simulink model "ex4_s1_simulink"  (R2014b)
settings: Solver=ode45  StartTime=0.0  StopTime=time  RelTol=1e-3
values from neighbouring files (symbols this model uses):
  C = 10e-6    (= 1e-05)    [ex4.m]
  G1 = 1/(R1*C*s + 1)    [ex4.m]
  R1 = 200    [ex4.m]
  R2 = 200    [ex4.m]
undefined symbols (not defined in the file or in its folder): S2
settings Model: Creator=gabras  LastModifiedBy=gabras

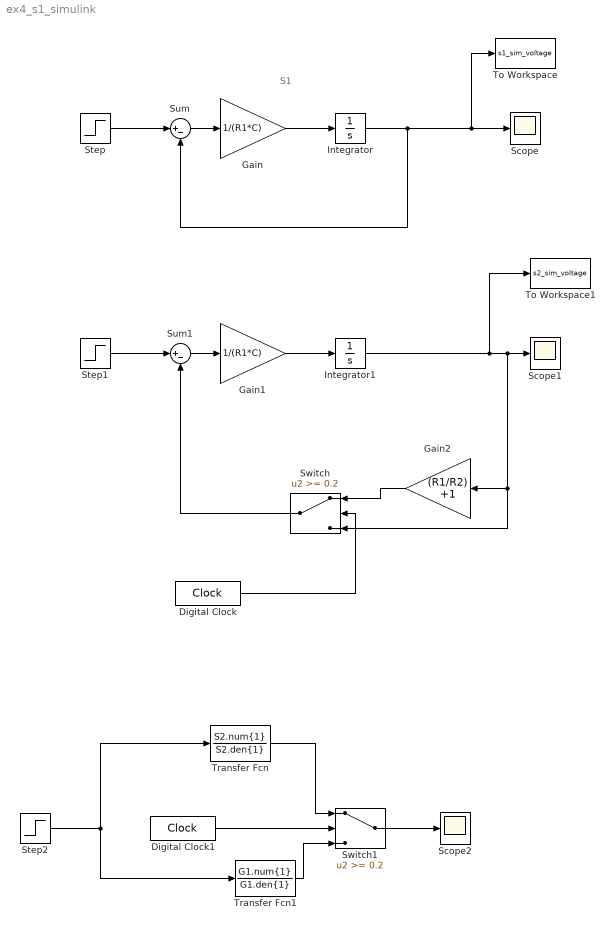
== system ex4_s1_simulink ==
  note: S1
  Digital Clock : DigitalClock  SampleTime=0.1
  Digital Clock1 : DigitalClock  SampleTime=0.1
  Gain : Gain  Gain=1/(R1*C)
  Gain1 : Gain  Gain=1/(R1*C)
  Gain2 : Gain  Gain=(R1/R2) +1
  Integrator : Integrator
  Integrator1 : Integrator
  Scope : Scope
  Scope1 : Scope
  Scope2 : Scope
      settings: SaveName=ScopeData2
  Step : Step  Time=0  After=12  SampleTime=0
  Step1 : Step  Time=0  After=12  SampleTime=0
  Step2 : Step  Time=0  After=12  SampleTime=0
  Sum : Sum  Inputs=|+-
  Sum1 : Sum  Inputs=|+-
  Switch : Switch  Threshold=0.2
  Switch1 : Switch  Threshold=0.2
  To Workspace : ToWorkspace  VariableName=s1_sim_voltage  SaveFormat=Timeseries  SampleTime=-1
  To Workspace1 : ToWorkspace  VariableName=s2_sim_voltage  SaveFormat=Timeseries  SampleTime=-1
  Transfer Fcn : TransferFcn  Numerator=S2.num{1}  Denominator=S2.den{1}
  Transfer Fcn1 : TransferFcn  Numerator=G1.num{1}  Denominator=G1.den{1}
  wires:
  Step/1 -> Sum/1
  Gain/1 -> Integrator/1
  Sum/1 -> Gain/1
  Integrator/1 -> Sum/2, To Workspace/1, Scope/1
  Digital Clock/1 -> Switch/2
  Gain2/1 -> Switch/1
  Step1/1 -> Sum1/1
  Gain1/1 -> Integrator1/1
  Sum1/1 -> Gain1/1
  Integrator1/1 -> To Workspace1/1, Switch/3, Gain2/1, Scope1/1
  Switch/1 -> Sum1/2
  Transfer Fcn/1 -> Switch1/1
  Transfer Fcn1/1 -> Switch1/3
  Digital Clock1/1 -> Switch1/2
  Step2/1 -> Transfer Fcn1/1, Transfer Fcn/1
  Switch1/1 -> Scope2/1
